simulink model "model1_panel"  (R2019b)
settings: Solver=VariableStepAuto  StartTime=0.0  StopTime=10.0  RelTol=1e-3
PreLoadFcn:
  | % Set physical parameters
  | panelMotorParams;
values from neighbouring files (symbols this model uses):
  J = m/12*(l^2*cos(beta)^2+d^2*sin(beta)^2+w^2)    [panelMotorParams.m]
  Kd = 5    [panelMotorParams.m]
settings Model: Creator=bneiswan  LastModifiedBy=bneiswan

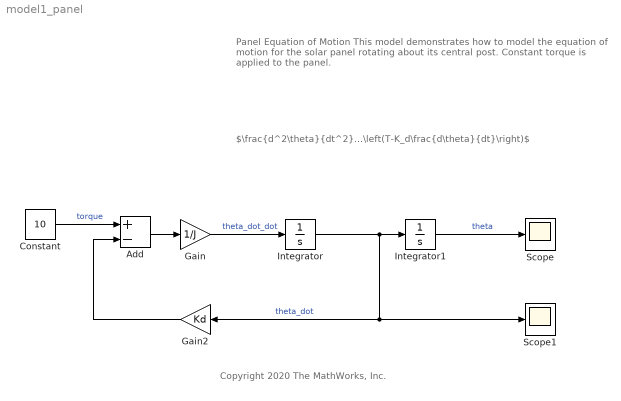
== system model1_panel ==
  note: Panel Equation of Motion
      |
      | This model demonstrates how to model the equation of motion for the solar panel rotating about its central post. Constant torque is applied to the panel.
  note: Copyright 2020 The MathWorks, Inc.
  note: $\frac{d^2\theta}{dt^2}=\frac{1}{J}\left(T-K_d\frac{d\theta}{dt}\right)$
  Add : Sum  Inputs=+-
  Constant : Constant  Value=10
  Gain : Gain  Gain=1/J
  Gain2 : Gain  Gain=Kd
  Integrator : Integrator
  Integrator1 : Integrator
  Scope : Scope
  Scope1 : Scope
  wires:
  Integrator1/1 -> Scope/1  "theta"
  Gain/1 -> Integrator/1  "theta_dot_dot"
  Integrator/1 -> Integrator1/1, Gain2/1, Scope1/1  "theta_dot"
  Constant/1 -> Add/1  "torque"
  Add/1 -> Gain/1
  Gain2/1 -> Add/2
